simulink model "RC_Circuit_ClosedLoop_Reference"  (R2023a)
settings: Solver=ode4  StartTime=0.0  StopTime=5  FixedStep=0.001  RelTol=1e-3
settings Model: Creator=Fasih  LastModifiedBy=Fasih

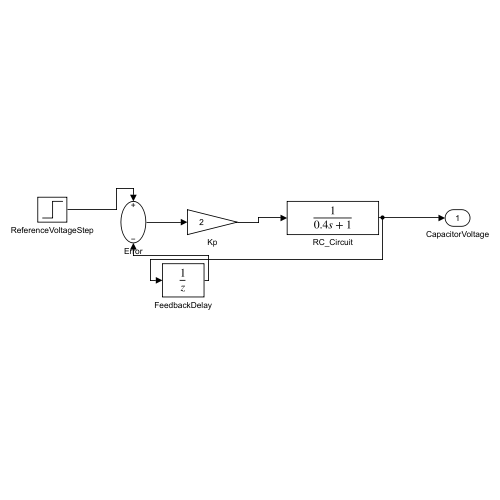
[thumbnail: Simulink's stored preview of the top-level diagram]
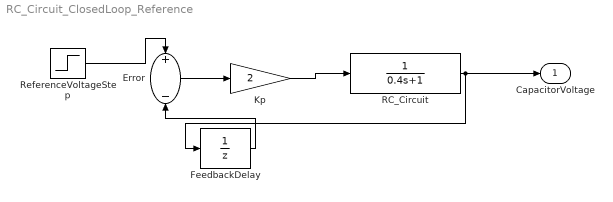
== system RC_Circuit_ClosedLoop_Reference ==
  Error : Sum  Inputs=+-
  FeedbackDelay : UnitDelay  SampleTime=0.001  HasFrameUpgradeWarning=on
  Kp : Gain  Gain=2
  RC_Circuit : TransferFcn  Numerator=1  Denominator=[0.4 1]
  ReferenceVoltageStep : Step  Time=0  SampleTime=0
  CapacitorVoltage : Outport
  wires:
  ReferenceVoltageStep/1 -> Error/1
  FeedbackDelay/1 -> Error/2
  Error/1 -> Kp/1
  Kp/1 -> RC_Circuit/1
  RC_Circuit/1 -> CapacitorVoltage/1, FeedbackDelay/1
